simulink model "L2c_mod"  (Simulink 7.0)
settings: Solver=ode45  StartTime=0.0  StopTime=10.0  RelTol=1e-3
undefined symbols (not defined in the file or in its folder): a, g, k, l, lam, m, ml
settings Model: Creator=Peter  LastModifiedBy=PeterSchmitz

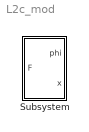
== system L2c_mod ==
  Subsystem : Subsystem

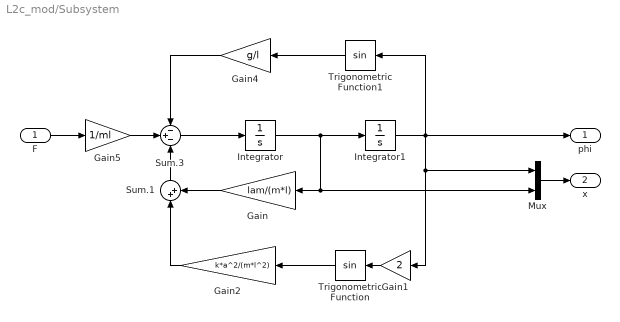
== system L2c_mod/Subsystem ==
  F : Inport
  Gain : Gain  Orientation=left  Gain=lam/(m*l)  ParameterDataType=sfix(16)  ParameterScaling=2^0  OutDataType=sfix(16)  OutScaling=2^0
  Gain1 : Gain  Orientation=left  Gain=2  ParameterDataType=sfix(16)  ParameterScaling=2^0  OutDataType=sfix(16)  OutScaling=2^0
  Gain2 : Gain  Orientation=left  Gain=k*a^2/(m*l^2)  ParameterDataType=sfix(16)  ParameterScaling=2^0  OutDataType=sfix(16)  OutScaling=2^0
  Gain4 : Gain  Orientation=left  Gain=g/l  ParameterDataType=sfix(16)  ParameterScaling=2^0  OutDataType=sfix(16)  OutScaling=2^0
  Gain5 : Gain  Gain=1/ml  ParameterDataType=sfix(16)  ParameterScaling=2^0  OutDataType=sfix(16)  OutScaling=2^0
  Integrator : Integrator
  Integrator1 : Integrator  LimitOutput=on  UpperSaturationLimit=pi/2  LowerSaturationLimit=-pi/2
  Mux : Mux  Inputs=2
  Sum.1 : Sum  Orientation=up  Inputs=|++  OutDataType=sfix(16)  OutScaling=2^0  SaturateOnIntegerOverflow=on  InputSameDT=on
  Sum.3 : Sum  Inputs=-+-  OutDataType=sfix(16)  OutScaling=2^0  SaturateOnIntegerOverflow=on  InputSameDT=on
  Trigonometric Function : Trigonometry  Orientation=left
  Trigonometric Function1 : Trigonometry  Orientation=left
  phi : Outport
  x : Outport  Port=2
  wires:
  Integrator/1 -> Integrator1/1, Mux/2, Gain/1
  Sum.3/1 -> Integrator/1
  Integrator1/1 -> Trigonometric Function1/1, phi/1, Mux/1, Gain1/1
  Gain/1 -> Sum.1/2
  Sum.1/1 -> Sum.3/3
  F/1 -> Gain5/1
  Trigonometric Function1/1 -> Gain4/1
  Gain4/1 -> Sum.3/1
  Gain5/1 -> Sum.3/2
  Mux/1 -> x/1
  Gain1/1 -> Trigonometric Function/1
  Trigonometric Function/1 -> Gain2/1
  Gain2/1 -> Sum.1/1
